simulink model "hnn_without_bias_with_cost_3_neurons"  (R2024b)
settings: Solver=VariableStepAuto  StartTime=0.0  StopTime=10.0  RelTol=1e-3
settings Model: Creator=merlin  LastModifiedBy=merlin

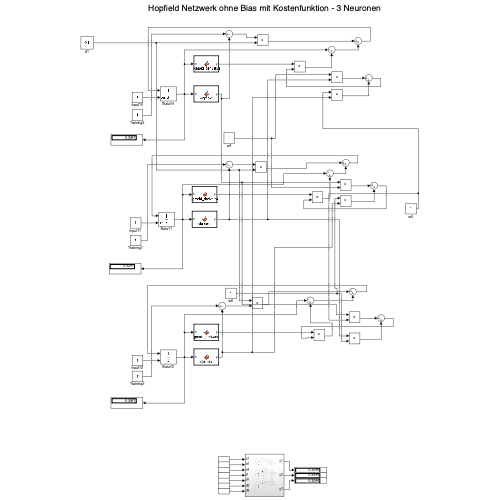
[thumbnail: Simulink's stored preview of the top-level diagram]
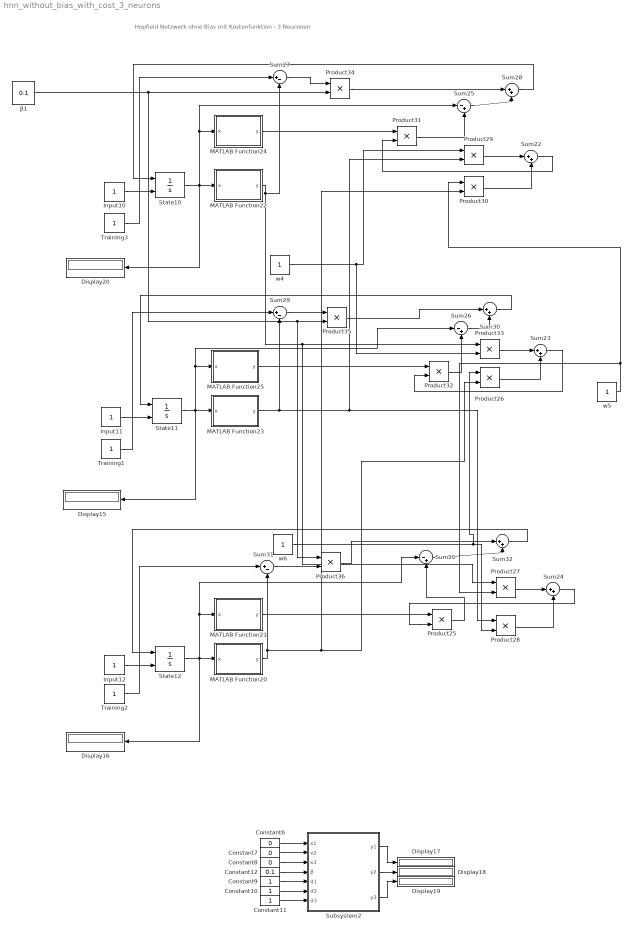
== system hnn_without_bias_with_cost_3_neurons ==
  note: Hopfield Netzwerk ohne Bias mit Kostenfunktion - 3 Neuronen
  Constant10 : Constant
  Constant11 : Constant
  Constant12 : Constant  Value=0.1
  Constant6 : Constant  Value=0
  Constant7 : Constant  Value=0
  Constant8 : Constant  Value=0
  Constant9 : Constant
  Display{15..20} (6 alike) : Display
  Input10 : Constant
  Input11 : Constant
  Input12 : Constant
  MATLAB Function20 : MATLAB Function  TreatAsAtomicUnit=on
  MATLAB Function21 : MATLAB Function  TreatAsAtomicUnit=on
  MATLAB Function22 : MATLAB Function  TreatAsAtomicUnit=on
  MATLAB Function23 : MATLAB Function  TreatAsAtomicUnit=on
  MATLAB Function24 : MATLAB Function  TreatAsAtomicUnit=on
  MATLAB Function25 : MATLAB Function  TreatAsAtomicUnit=on
  Product{25..36} (12 alike) : Product
  State10 : Integrator  InitialConditionSource=external
  State11 : Integrator  InitialConditionSource=external
  State12 : Integrator  InitialConditionSource=external
  Subsystem2 : Subsystem
  Sum20 : Sum  Inputs=|-+
  Sum{22..24,28,30,32} (6 alike) : Sum  Inputs=|++
  Sum25 : Sum  Inputs=|-+
  Sum26 : Sum  Inputs=|-+
  Sum27 : Sum  Inputs=|+-
  Sum29 : Sum  Inputs=|+-
  Sum31 : Sum  Inputs=|+-
  Training1 : Constant
  Training2 : Constant
  Training3 : Constant
  w4 : Constant
  w5 : Constant
  w6 : Constant
  β1 : Constant  Value=0.1  VectorParams1D=off
  wires:
  Training2/1 -> Sum31/1
  w5/1 -> Product27/2, Product30/1
  Product36/1 -> Sum32/1
  MATLAB Function21/1(y) -> Product25/1
  Sum32/1 -> State12/1
  Product32/1 -> Sum26/2
  Subsystem2/3(y3) -> Display19/1
  Product27/1 -> Sum24/1
  Sum30/1 -> State11/1
  Input12/1 -> State12/2
  Sum28/1 -> State10/1
  β1/1 -> Product36/1, Product35/2, Product34/2
  Product29/1 -> Sum22/1
  Product35/1 -> Sum30/1
  MATLAB Function23/1(y) -> Product28/1, Product29/2, Sum29/2
  Product31/1 -> Sum25/2
  Sum29/1 -> Product35/1
  State10/1 -> Display20/1, Sum25/1, MATLAB Function24/1(x), MATLAB Function22/1(x)
  Product34/1 -> Sum28/1
  Constant11/1 -> Subsystem2/7(d3)
  Constant10/1 -> Subsystem2/6(d2)
  Product26/1 -> Sum23/2
  Sum25/1 -> Sum28/2
  State12/1 -> Display16/1, Sum20/1, MATLAB Function21/1(x), MATLAB Function20/1(x)
  Product28/1 -> Sum24/2
  Sum20/1 -> Sum32/2
  Product33/1 -> Sum23/1
  Constant12/1 -> Subsystem2/4(β)
  Input11/1 -> State11/2
  w6/1 -> Product28/2, Product26/1
  Sum23/1 -> Product32/2
  Constant9/1 -> Subsystem2/5(d1)
  Sum22/1 -> Product31/2
  Constant7/1 -> Subsystem2/2(x2)
  Input10/1 -> State10/2
  State11/1 -> Display15/1, Sum26/1, MATLAB Function25/1(x), MATLAB Function23/1(x)
  Training1/1 -> Sum29/1
  MATLAB Function24/1(y) -> Product31/1
  Training3/1 -> Sum27/1
  Subsystem2/2(y2) -> Display18/1
  MATLAB Function25/1(y) -> Product32/1
  Sum24/1 -> Product25/2
  Sum27/1 -> Product34/1
  Constant6/1 -> Subsystem2/1(x1)
  MATLAB Function20/1(y) -> Product26/2, Product30/2, Sum31/2
  Sum26/1 -> Sum30/2
  Constant8/1 -> Subsystem2/3(x3)
  Sum31/1 -> Product36/2
  w4/1 -> Product33/2, Product29/1
  Product30/1 -> Sum22/2
  MATLAB Function22/1(y) -> Sum27/2, Product27/1, Product33/1
  Subsystem2/1(y1) -> Display17/1
  Product25/1 -> Sum20/2

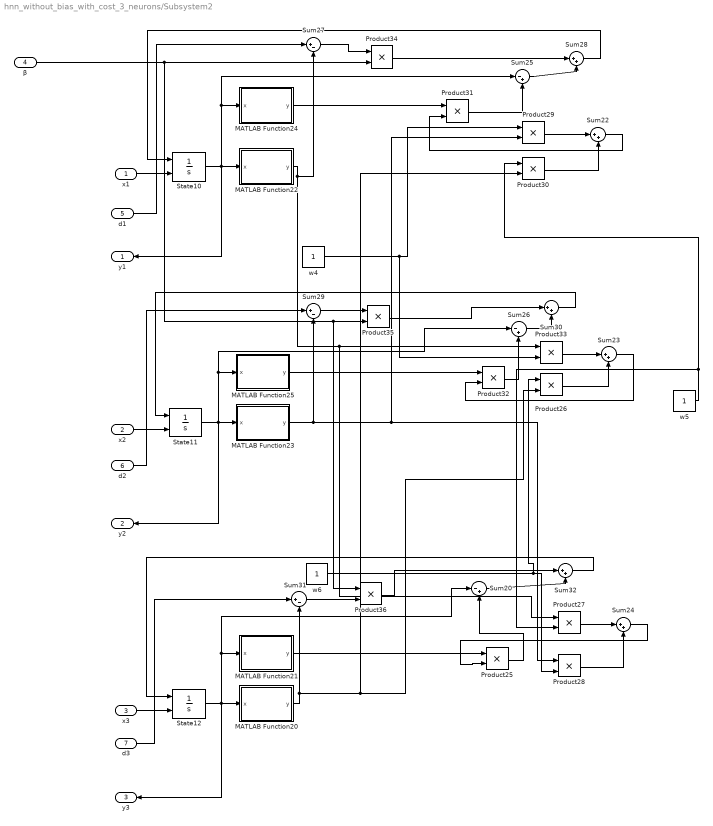
== system hnn_without_bias_with_cost_3_neurons/Subsystem2 ==
  x1 : Inport
  x2 : Inport  Port=2
  x3 : Inport  Port=3
  β : Inport  Port=4
  d1 : Inport  Port=5
  d2 : Inport  Port=6
  d3 : Inport  Port=7
  MATLAB Function20 : MATLAB Function  TreatAsAtomicUnit=on
  MATLAB Function21 : MATLAB Function  TreatAsAtomicUnit=on
  MATLAB Function22 : MATLAB Function  TreatAsAtomicUnit=on
  MATLAB Function23 : MATLAB Function  TreatAsAtomicUnit=on
  MATLAB Function24 : MATLAB Function  TreatAsAtomicUnit=on
  MATLAB Function25 : MATLAB Function  TreatAsAtomicUnit=on
  Product{25..36} (12 alike) : Product
  State10 : Integrator  InitialConditionSource=external
  State11 : Integrator  InitialConditionSource=external
  State12 : Integrator  InitialConditionSource=external
  Sum20 : Sum  Inputs=|-+
  Sum{22..24,28,30,32} (6 alike) : Sum  Inputs=|++
  Sum25 : Sum  Inputs=|-+
  Sum26 : Sum  Inputs=|-+
  Sum27 : Sum  Inputs=|+-
  Sum29 : Sum  Inputs=|+-
  Sum31 : Sum  Inputs=|+-
  w4 : Constant
  w5 : Constant
  w6 : Constant
  y1 : Outport
  y2 : Outport  Port=2
  y3 : Outport  Port=3
  wires:
  d2/1 -> Sum29/1
  d3/1 -> Sum31/1
  State11/1 -> y2/1, Sum26/1, MATLAB Function25/1(x), MATLAB Function23/1(x)
  x3/1 -> State12/2
  Product27/1 -> Sum24/1
  MATLAB Function22/1(y) -> Sum27/2, Product27/1, Product33/1
  Product28/1 -> Sum24/2
  w6/1 -> Product28/2, Product26/1
  Product26/1 -> Sum23/2
  Sum25/1 -> Sum28/2
  w5/1 -> Product27/2, Product30/1
  Product33/1 -> Sum23/1
  x2/1 -> State11/2
  Product36/1 -> Sum32/1
  MATLAB Function24/1(y) -> Product31/1
  MATLAB Function20/1(y) -> Product26/2, Product30/2, Sum31/2
  State10/1 -> y1/1, Sum25/1, MATLAB Function24/1(x), MATLAB Function22/1(x)
  Product25/1 -> Sum20/2
  x1/1 -> State10/2
  Sum20/1 -> Sum32/2
  MATLAB Function21/1(y) -> Product25/1
  Product34/1 -> Sum28/1
  Sum29/1 -> Product35/1
  Sum28/1 -> State10/1
  Product31/1 -> Sum25/2
  Sum22/1 -> Product31/2
  Sum23/1 -> Product32/2
  Sum31/1 -> Product36/2
  State12/1 -> y3/1, Sum20/1, MATLAB Function21/1(x), MATLAB Function20/1(x)
  Sum24/1 -> Product25/2
  Sum32/1 -> State12/1
  w4/1 -> Product33/2, Product29/1
  MATLAB Function25/1(y) -> Product32/1
  β/1 -> Product36/1, Product35/2, Product34/2
  MATLAB Function23/1(y) -> Product28/1, Product29/2, Sum29/2
  Product30/1 -> Sum22/2
  Product29/1 -> Sum22/1
  Sum27/1 -> Product34/1
  Sum26/1 -> Sum30/2
  Product32/1 -> Sum26/2
  Product35/1 -> Sum30/1
  Sum30/1 -> State11/1
  d1/1 -> Sum27/1

== matlab function hnn_without_bias_with_cost_3_neurons/MATLAB Function21 ==
  data: x input; y output
function y = sigmoid_derivative(x)
sigmoid = 1 ./ (1 + exp(-x));
y = sigmoid .* (1 - sigmoid);
end

== matlab function hnn_without_bias_with_cost_3_neurons/MATLAB Function22 ==
  data: x input; y output
function y = sigmoid(x)
y = 1 ./ (1 + exp(-x));
end

== matlab function hnn_without_bias_with_cost_3_neurons/MATLAB Function23 ==
  data: x input; y output
function y = sigmoid(x)
y = 1 ./ (1 + exp(-x));
end

== matlab function hnn_without_bias_with_cost_3_neurons/MATLAB Function24 ==
  data: x input; y output
function y = sigmoid_derivative(x)
sigmoid = 1 ./ (1 + exp(-x));
y = sigmoid .* (1 - sigmoid);
end

== matlab function hnn_without_bias_with_cost_3_neurons/MATLAB Function25 ==
  data: x input; y output
function y = sigmoid_derivative(x)
sigmoid = 1 ./ (1 + exp(-x));
y = sigmoid .* (1 - sigmoid);
end

== matlab function hnn_without_bias_with_cost_3_neurons/Subsystem2/MATLAB Function20 ==
  data: x input; y output
function y = sigmoid(x)
y = 1 ./ (1 + exp(-x));
end

== matlab function hnn_without_bias_with_cost_3_neurons/Subsystem2/MATLAB Function21 ==
  data: x input; y output
function y = sigmoid_derivative(x)
sigmoid = 1 ./ (1 + exp(-x));
y = sigmoid .* (1 - sigmoid);
end

== matlab function hnn_without_bias_with_cost_3_neurons/Subsystem2/MATLAB Function22 ==
  data: x input; y output
function y = sigmoid(x)
y = 1 ./ (1 + exp(-x));
end

== matlab function hnn_without_bias_with_cost_3_neurons/MATLAB Function20 ==
  data: x input; y output
function y = sigmoid(x)
y = 1 ./ (1 + exp(-x));
end

== matlab function hnn_without_bias_with_cost_3_neurons/Subsystem2/MATLAB Function23 ==
  data: x input; y output
function y = sigmoid(x)
y = 1 ./ (1 + exp(-x));
end

== matlab function hnn_without_bias_with_cost_3_neurons/Subsystem2/MATLAB Function24 ==
  data: x input; y output
function y = sigmoid_derivative(x)
sigmoid = 1 ./ (1 + exp(-x));
y = sigmoid .* (1 - sigmoid);
end

== matlab function hnn_without_bias_with_cost_3_neurons/Subsystem2/MATLAB Function25 ==
  data: x input; y output
function y = sigmoid_derivative(x)
sigmoid = 1 ./ (1 + exp(-x));
y = sigmoid .* (1 - sigmoid);
end
